simulink model "normalOperations"  (R2022a)
settings: Solver=VariableStepAuto  StartTime=0.0  StopTime=10.0  RelTol=1e-3
settings Model: Creator=Nate  LastModifiedBy=Nate
settings DebuggingCC: UnconnectedInputMsg=warning  UnconnectedOutputMsg=warning  UnconnectedLineMsg=warning
settings RTWCC: DLArmComputeVersion=19.05

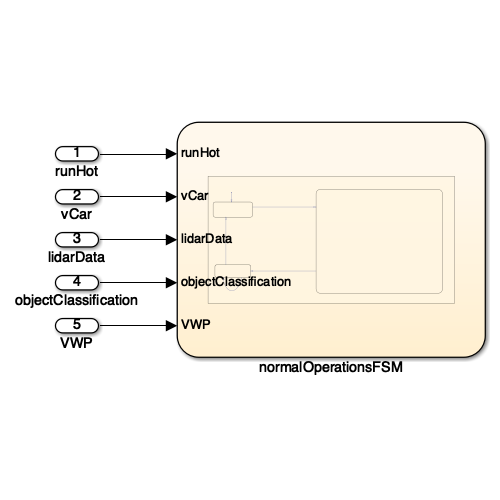
[thumbnail: Simulink's stored preview of the top-level diagram]
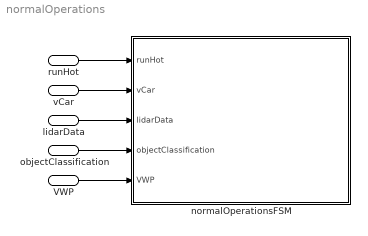
== system normalOperations ==
  runHot : Inport
  vCar : Inport  Port=2
  lidarData : Inport  Port=3
  objectClassification : Inport  Port=4
  VWP : Inport  Port=5
  normalOperationsFSM : Stateflow chart  TreatAsAtomicUnit=on
  wires:
  runHot/1 -> normalOperationsFSM/1(runHot)
  vCar/1 -> normalOperationsFSM/2(vCar)
  lidarData/1 -> normalOperationsFSM/3(lidarData)
  objectClassification/1 -> normalOperationsFSM/4(objectClassification)
  VWP/1 -> normalOperationsFSM/5(VWP)

== stateflow chart normalOperations/normalOperationsFSM ==
  state normalOperations [group]
    state autonomous_mode
      en: normalOpState = 1
      du:
      updateObstaclesInProjectedOccupancyZones(ActiveObjectList, VWP, ...
      objectClassification, lidarData)
      du:
      curObject = sort(ActiveObjectList)
      du:
      SubMachineRunning = StopSignEnable || VariableStopEnable || ReroutingEnable
      if curObject == None
      disp("curObject is None")
      elseif  curObject == stopSign
      StopSignEnable = true
      VariableStopEnable = false
      ReroutingEnable = false
      elseif curObject == stopLight || RR || movingObstacle
      StopSignEnable = false
      VariableStopEnable = true
      ReroutingEnable = false
      else
      StopSignEnable = false
      VariableStopEnable = false
      ReroutingEnable = true
      end
      du:
      if SubMachineRunning == false && abs(vCar - lastSeenSpeedLimit) > 0.5
      SpeedChangeEnable = true
      end
    state manual_mode
      en: normalOpState = 0
      en: ActiveObjectList = []
    state wait_for_stopped
      en: normalOpState = 2
    (default) -> manual_mode
    manual_mode -> autonomous_mode : [runHot == true && VWP.length > 0]
    wait_for_stopped -> manual_mode [order 1] : [vCar == 0]
    autonomous_mode -> wait_for_stopped : [VWP.length == 0]
        | {updateVWP(distance,VWP)}
    wait_for_stopped -> wait_for_stopped [order 2]
  data: distance local; updateVWP local; runHot input; movingObstacle constant double; stopLight constant double; stopSign constant double; None constant double; vCar input; lidarData input; updateObstaclesInProjectedOccupancyZones local; objectClassification input; normalOpState local; SpeedChangeEnable local; ReroutingEnable local; curObject local; StopSignEnable local; ActiveObjectList local; VariableStopEnable local; SubMachineRunning local; VWP input; RR constant double
